simulink library "Pump_Const"  (R2016b)
settings: Solver=ode45  StartTime=0.0  StopTime=10.0  RelTol=1e-3  EnableMultiTasking=on
undefined symbols (not defined in the file): Water
libraries: carnot x2
settings Model: Creator=lena.frank  LastModifiedBy=drhf
settings DataIOCC: LimitDataPoints=on  SaveFormat=Array  SignalLoggingSaveFormat=ModelDataLogs
settings OptimizationCC: ExpressionDepthLimit=2147483647  LifeSpan=inf
settings DebuggingCC: UnderspecifiedInitializationDetection=Classic  MergeDetectMultiDrivingBlocksExec=none  SolverPrmCheckMsg=warning  FcnCallInpInsideContextMsg=warning  StateNameClashWarn=warning  SFUnexpectedBacktrackingDiag=warning  SFNoUnconditionalDefaultTransitionDiag=warning  SFExecutionAtInitializationDiag=none
settings HardwareCC: ProdBitPerPointer=32  ProdBitPerSizeT=32  ProdBitPerPtrDiffT=32  ProdLargestAtomicFloat=None  ProdIntDivRoundTo=Undefined  ProdEndianess=Unspecified  ProdWordSize=32  ProdHWDeviceType=32-bit Generic
settings ModelReferenceCC: PropagateSignalLabelsOutOfModel=off
settings GRTTargetCC: TargetLangStandard=C89/C90 (ANSI)  GeneratePreprocessorConditionals=Disable all  CombineOutputUpdateFcns=off  GRTInterface=on
settings ConfigComp: CovMetricSettings=dw  CovHtmlReporting=on  CovSaveCumulativeToWorkspaceVar=on  CovSaveSingleToWorkspaceVar=on  CovExternalEMLEnable=off

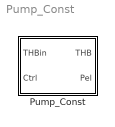
== system Pump_Const ==
  Pump_Const : Subsystem  mask(constant pump){mdotmax=1200/3600, dia=0.025, power=30, p0=2e5, fluid_id=Water, mix=0, mix2=0, mix3=0, UA=1, mcp=4200, tamb=20, cp_approx=4000}
      mask prompts: mdotmax "massflow rate [kg/s]"; dia "diameter at in- and outlet [m]"; power "electric power consumption [W]"; p0 "system pressure [Pa]"; fluid_id "fluid"; mix "percentage of fluid mix [0..1]"; mix2 "fluid mixture 2 [0..1]"; mix3 "fluid mixture 3 [0..1]"; UA "Thermal loss coefficient to ambient in W/K"; mcp "Thermal capacity in J/K"; tamb "Ambient temperature for losses in °C"; cp_approx "heat capacity of fluid in J/kg/K (approximate value for thermal inertia)"
      mask help:
      | Set constant massflow rate according to the control signal.
      | The pump has a thermal capacity and losses to ambient.
      mask Help: web(fullfile(path_carnot('help'),'Pump_Const.html'),'-helpbrowser')
      mask TypeOptions mdotmax: Pump_basic/mdotmax
      mask TypeOptions dia: Pump_basic/dia
      mask TypeOptions power: Pump_basic/power
      mask TypeOptions p0: Pump_basic/p0
      mask TypeOptions fluid_id: Pump_basic/fluid_id
      mask TypeOptions mix: Pump_basic/mix
      mask TypeOptions mix2: Pump_basic/mix2
      mask TypeOptions mix3: Pump_basic/mix3
      mask TypeOptions UA: Thermal_Capacity/UA
      mask TypeOptions mcp: Thermal_Capacity/mcp
      mask TypeOptions tamb: Thermal_Capacity/Tamb
      mask TypeOptions cp_approx: Thermal_Capacity/cp_approx
      mask Display:
      | plot(0,0,100,100,[40,70,40,30,30,40,60,70,70,60,40],[70,50,30,40,60,70,70,60,40,30,30])
      | % port_label('input',1,'THB')
      | % port_label('input',2,'ctr')
      | % port_label('output',1,'THB')
      | % port_label('output',2,'Pel')

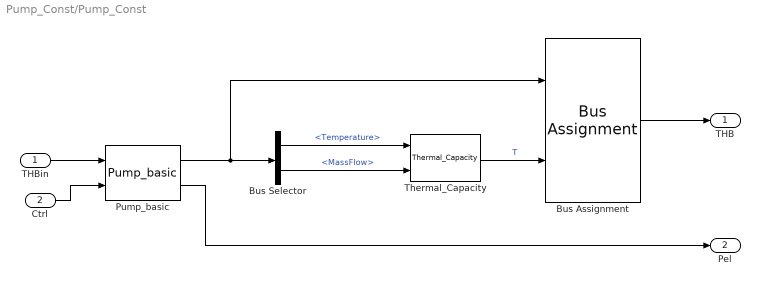
== system Pump_Const/Pump_Const ==
  THBin : Inport
  Ctrl : Inport  Port=2
  Bus Assignment : BusAssignment  AssignedSignals=Temperature
  Bus Selector : BusSelector  OutputSignals=Temperature,MassFlow
  Pump_basic : carnot/Basic/Hydraulics/Pump_basic  mdotmax=mdotmax  fluid_id=Water  mix=mix  mix2=mix2  mix3=mix3  power=power  p0=p0  dia=dia  ID=No Pressure Drop  hgt=0
  Thermal_Capacity : carnot/Basic/Thermal_Models/Thermal_Capacity  UA=UA  mcp=mcp  Tamb=tamb  cp_approx=cp_approx
  THB : Outport
  Pel : Outport  Port=2
  wires:
  Bus Assignment/1 -> THB/1
  Pump_basic/2 -> Pel/1
  Bus Selector/2 -> Thermal_Capacity/2  "<MassFlow>"
  Ctrl/1 -> Pump_basic/2
  Thermal_Capacity/1 -> Bus Assignment/2  "T"
  Bus Selector/1 -> Thermal_Capacity/1  "<Temperature>"
  THBin/1 -> Pump_basic/1
  Pump_basic/1 -> Bus Selector/1, Bus Assignment/1
